simulink model "Unicycle_kinematic_model"  (R2024b)
settings: Solver=VariableStepAuto  StartTime=0.0  StopTime=10.0  RelTol=1e-3
libraries: simulink_extras x1
settings Model: Creator=Nabil  LastModifiedBy=Nabil

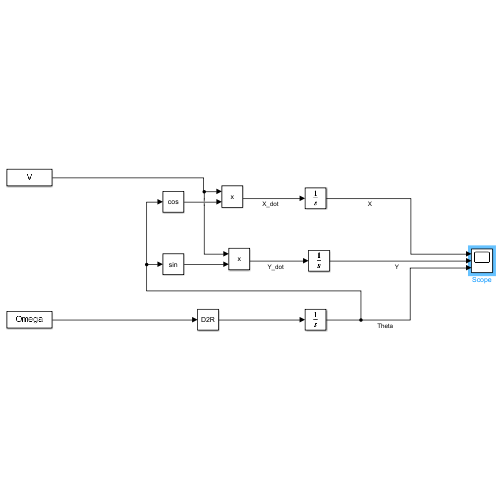
[thumbnail: Simulink's stored preview of the top-level diagram]
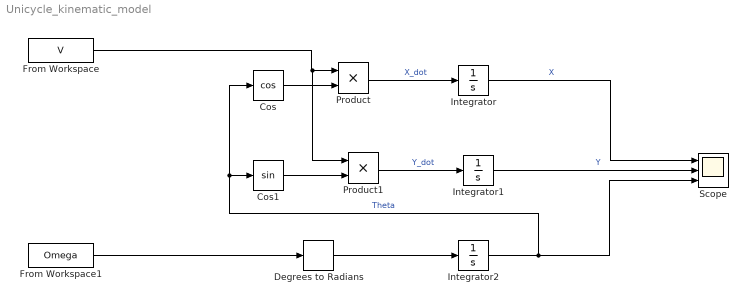
== system Unicycle_kinematic_model ==
  Cos : Trigonometry  Operator=cos
  Cos1 : Trigonometry
  Degrees to Radians : simulink_extras/Transformations/Degrees to Radians
  From Workspace : FromWorkspace  VariableName=V
  From Workspace1 : FromWorkspace  VariableName=Omega
  Integrator : Integrator
  Integrator1 : Integrator
  Integrator2 : Integrator
  Product : Product
  Product1 : Product
  Scope : Scope  NumInputPorts=3
  wires:
  Integrator1/1 -> Scope/2  "Y"
  Integrator/1 -> Scope/1  "X"
  Integrator2/1 -> Cos/1, Cos1/1, Scope/3  "Theta"
  From Workspace1/1 -> Degrees to Radians/1
  Product/1 -> Integrator/1  "X_dot"
  Product1/1 -> Integrator1/1  "Y_dot"
  Degrees to Radians/1 -> Integrator2/1
  Cos/1 -> Product/2
  From Workspace/1 -> Product1/1, Product/1
  Cos1/1 -> Product1/2
